simulink model "Mining_Loader_Sweep"  (R2026a)
settings: Solver=ode23t  StopTime=stopTime  AbsTol=1e-3
PostLoadFcn:
  | [extInput_Mining_Loader_Sweep, minMachParams, Init] = test_MLSweep_braking('Mining_Loader_Sweep',minMachParams,testSettings,Init,5,0,0,0,0,0,40);
undefined symbols (not defined in the file): bucketLoadMass, minMachParams, targetSpeedMag, testSettings
libraries: sm_mining_loader_lib x1, simulink_extras x1
settings Model: Creator=gabri  LastModifiedBy=smiller
settings SolverCC: MaxConsecutiveMinStep=5
settings DataIOCC: ExternalInput=extInput_Mining_Loader_Sweep  LoadExternalInput=on  SignalLoggingName=logsout_Mining_Loader_Sweep
settings DebuggingCC: AlgebraicLoopMsg=error
settings SimscapeCC: SimscapeNominalValues="[{\"value\":\"1\",\"unit\":\"A\"},{\"value\":\"1\",\"unit\":\"bar\"},{\"value\":\"1\",\"unit\":\"cm^2\"},{\"value\":\"1\",\"unit\":\"cm^3/s\"},{\"value\":\"1\",\"unit\":\"kJ/kg\"},{\"value\":\"1\",\"unit\":\"kW\"},{\"value\":\"1\",\"unit\":\"l\"},{\"value\":\"1\",\"unit\":\"N\"},{\"value\":\"1\",\"unit\":\"N*m\"},{\"value\":\"1\",\"unit\":\"V\"}]"  SimscapeLogName=simlog_Mining_Loader_Sweep  SimscapeLogLimitData=off  SimscapeLogDataHistory=5000.0
settings DiagnosticsConfigSet: SimMechanicsConflictingReferenceFrames=none
settings ExplorerConfigSet: InternalSimMechanicsExplorerSettings="<ExplorerConfiguration><canonicalview>default</canonicalview><TilePanel><TileInfo><Tiles Columns=\"1\" Count=\"1\" Height=\"438\" Rows=\"1\" Width=\"828\"><Row Weight=\"1\"/><Column Weight=\"1\"/><Tile Height=\"1\" Width=\"1\" X=\"0\" Y=\"0\"/></Tiles></TileInfo><SceneInfo><SceneViewer><IsThisViewStd><IsStandardView>off</IsStandardView><StandardViewName>Front</StandardViewName></IsThisViewStd><BGColor><R>1</R><G>1</G><B>1</B><A>1</A></BGColor><Camera><DoPerspective>on</DoPerspective><Position><X>-19.655173879230539</X><Y>-9.0222687540439601</Y><Z>-1.8989073435199815</Z></Position><Center><X>-19.622924303554189</X><Y>-8.0228109525652247</Y><Z>-1.892268975347827</Z></Center><Up><X>-0.00021408927402311921</X><Y>-0.0066349150538512255</Y><Z>0.99997796579125231</Z></Up><XLim>0.46630765815499881</XLim><YLim>0.46630765815499881</YLim><ViewLimDist>0.01</ViewLimDist></Camera></SceneViewer></SceneInfo></TilePanel><MechEditorPanel><GfxPanelCameraMap><MapElement CameraMLId=\"Camera10\" GfxPanelIndex=\"0\"/></GfxPanelCameraMap><Cameras><Camera><Id>Camera1</Id><Value><Name>Track LR</Name><NativeCamera><PositionTrackingFeature>Mining_Loader.Vehicle.Camera_Frames_R.Cam_Ref_LR.R</PositionTrackingFeature><CenterTrackingFeature>Mining_Loader.Vehicle.Camera_Frames_R.Cam_Ref_Ctr.R</CenterTrackingFeature><UpVectorTrackingFeature>Mining_Loader.World_Frame.W</UpVectorTrackingFeature><CenterTrackingOrigin>on</CenterTrackingOrigin><UpVectorTrackingDirection>+Z</UpVectorTrackingDirection></NativeCamera></Value></Camera><Camera><Id>Camera2</Id><Value><Name>Track RR</Name><NativeCamera><PositionTrackingFeature>Mining_Loader.Vehicle.Camera_Frames_R.Cam_Ref_RR.R</PositionTrackingFeature><CenterTrackingFeature>Mining_Loader.Vehicle.Camera_Frames_R.Cam_Ref_Ctr.R</CenterTrackingFeature><UpVectorTrackingFeature>Mining_Loader.World_Frame.W</UpVectorTrackingFeature><CenterTrackingOrigin>on</CenterTrackingOrigin><UpVectorTrackingDirection>+Z</UpVectorTrackingDirection></NativeCamera></Value></Camera><Camera><Id>Camera3</Id><Value><Name>Track FL</Name><NativeCamera><PositionTrackingFeature>Mining_Loader.Vehicle.Camera_Frames_F.Cam_Ref_FL.R</PositionTrackingFeature><CenterTrackingFeature>Mining_Loader.Vehicle.Camera_Frames_F.Cam_Ref_Ctr.R</CenterTrackingFeature><UpVectorTrackingFeature>Mining_Loader.World_Frame.W</UpVectorTrackingFeature><CenterTrackingOrigin>on</CenterTrackingOrigin><UpVectorTrackingDirection>+Z</UpVectorTrackingDirection></NativeCamera></Value></Camera><Camera><Id>Camera4</Id><Value><Name>Track FR</Name><NativeCamera><PositionTrackingFeature>Mining_Loader.Vehicle.Camera_Frames_F.Cam_Ref_FR.R</PositionTrackingFeature><CenterTrackingFeature>Mining_Loader.Vehicle.Camera_Frames_F.Cam_Ref_Ctr.R</CenterTrackingFeature><UpVectorTrackingFeature>Mining_Loader.World_Frame.W</UpVectorTrackingFeature><CenterTrackingOrigin>on</CenterTrackingOrigin><UpVectorTrackingDirection>+Z</UpVectorTrackingDirection></NativeCamera></Value></Camera><Camera><Id>Camera5</Id><Value><Name>Track Frame Right</Name><NativeCamera><PositionTrackingFeature>Mining_Loader.Vehicle.Camera_Frames_F.Cam_Ref_Right.R</PositionTrackingFeature><CenterTrackingFeature>Mining_Loader.Vehicle.Camera_Frames_F.Cam_Ref_Right.R</CenterTrackingFeature><UpVectorTrackingFeature>Mining_Loader.World_Frame.W</UpVectorTrackingFeature><CenterTrackingOrigin>off</CenterTrackingOrigin><CenterTrackingDirection>-Y</CenterTrackingDirection><UpVectorTrackingDirection>+Z</UpVectorTrackingDirection></NativeCamera></Value></Camera><Camera><Id>Camera6</Id><Value><Name>Track Frame Left</Name><NativeCamera><PositionTrackingFeature>Mining_Loader.Vehicle.Camera_Frames_F.Cam_Ref_Left.R</PositionTrackingFeature><CenterTrackingFeature>Mining_Loader.Vehicle.Camera_Frames_F.Cam_Ref_Left.R</CenterTrackingFeature><UpVectorTrackingFeature>Mining_Loader.World_Frame.W</UpVectorTrackingFeature><CenterTrackingOrigin>off</CenterTrackingOrigin><CenterTrackingDirection>+Y</CenterTrackingDirection><UpVectorTrackingDirection>+Z</UpVectorTrackingDirection></NativeCamera></Value></Camera><Camera><Id>Camera7</Id><Value><Name>Track Frame Top Down</Name><NativeCamera><PositionTrackingFeature>Mining_Loader.Vehicle.Camera_Frames_F.Cam_Ref_Top_Down.R</PositionTrackingFeature><CenterTrackingFeature>Mining_Loader.Vehicle.Camera_Frames_F.Cam_Ref_Top_Down.R</CenterTrackingFeature><UpVectorTrackingFeature>Mining_Loader.Vehicle.Camera_Frames_F.Cam_Ref_Top_Down.R</UpVectorTrackingFeature><CenterTrackingOrigin>off</CenterTrackingOrigin><CenterTrackingDirection>-Z</CenterTrackingDirection><UpVectorTrackingDirection>+Y</UpVectorTrackingDirection></NativeCamera></Value></Camera><Camera><Id>Camera8</Id><Value><Name>Track Frame Rear Fwd</Name><NativeCamera><PositionTrackingFeature>Mining_Loader.Vehicle.Camera_Frames_F.Cam_Ref_Top_Rear_Fwd.R</PositionTrackingFeature><CenterTrackingFeature>Mining_Loader.Vehicle.Camera_Frames_F.Cam_Ref_Top_Rear_Fwd.R</CenterTrackingFeature><UpVectorTrackingFeature>Mining_Loader.World_Frame.W</UpVectorTrackingFeature><CenterTrackingOrigin>off</CenterTrackingOrigin><CenterTrackingDirection>+X</CenterTrackingDirection><UpVectorTrackingDirection>+Z</UpVectorTrackingDirection></NativeCamera></Value></Camera><Camera><Id>Camera9</Id><Value><Name>Track Chassis Right</Name><NativeCamera><PositionTrackingFeature>Mining_Loader.Vehicle.Camera_Frames_R.Cam_Ref_Right.R</PositionTrackingFeature><CenterTrackingFeature>Mining_Loader.Vehicle.Camera_Frames_R.Cam_Ref_Right.R</CenterTrackingFeature><UpVectorTrackingFeature>Mining_Loader.World_Frame.W</UpVectorTrackingFeature><CenterTrackingOrigin>off</CenterTrackingOrigin><CenterTrackingDirection>-Y</CenterTrackingDirection><UpVectorTrackingDirection>+Z</UpVectorTrackingDirection></NativeCamera></Value></Camera><Camera><Id>Camera10</Id><Value><Name>Track Chassis Left</Name><NativeCamera><PositionTrackingFeature>Mining_Loader.Vehicle.Camera_Frames_F.Cam_Ref_Left.R</PositionTrackingFeature><CenterTrackingFeature>Mining_Loader.Vehicle.Camera_Frames_F.Cam_Ref_Left.R</CenterTrackingFeature><UpVectorTrackingFeature>Mining_Loader.World_Frame.W</UpVectorTrackingFeature><CenterTrackingOrigin>off</CenterTrackingOrigin><CenterTrackingDirection>+Y</CenterTrackingDirection><UpVectorTrackingDirection>+Z</UpVectorTrackingDirection></NativeCamera></Value></Camera><Camera><Id>Camera11</Id><Value><Name>Track Chassis Top Down</Name><NativeCamera><PositionTrackingFeature>Mining_Loader.Vehicle.Camera_Frames_R.Cam_Ref_Top_Down.R</PositionTrackingFeature><CenterTrackingFeature>Mining_Loader.Vehicle.Camera_Frames_R.Cam_Ref_Top_Down.R</CenterTrackingFeature><UpVectorTrackingFeature>Mining_Loader.Vehicle.Camera_Frames_R.Cam_Ref_Top_Down.R</UpVectorTrackingFeature><CenterTrackingOrigin>off</CenterTrackingOrigin><CenterTrackingDirection>-Z</CenterTrackingDirection><UpVectorTrackingDirection>+Y</UpVectorTrackingDirection></NativeCamera></Value></Camera><Camera><Id>Camera12</Id><Value><Name>Track Chassis Rear Fwd</Name><NativeCamera><PositionTrackingFeature>Mining_Loader.Vehicle.Camera_Frames_R.Cam_Ref_Top_Rear_Fwd.R</PositionTrackingFeature><CenterTrackingFeature>Mining_Loader.Vehicle.Camera_Frames_R.Cam_Ref_Top_Rear_Fwd.R</CenterTrackingFeature><UpVectorTrackingFeature>Mining_Loader.World_Frame.W</UpVectorTrackingFeature><CenterTrackingOrigin>off</CenterTrackingOrigin><CenterTrackingDirection>+X</CenterTrackingDirection><UpVectorTrackingDirection>+Z</UpVectorTrackingDirection></NativeCamera></Value></Camera></Cameras><VideoCreator><IncludeTiles>All</IncludeTiles><IncludeTime>on</IncludeTime><IncludeWorldFrame>off</IncludeWorldFrame><PlaybackSpeedRatio>1</PlaybackSpeedRatio><FrameRate>30</FrameRate><FrameSize>auto</FrameSize><VideoFormat>UncompressedAVI</VideoFormat></VideoCreator></MechEditorPanel><PlaybackSettings><PlaybackSpeedFactor>8</PlaybackSpeedFactor></PlaybackSettings></ExplorerConfiguration>"

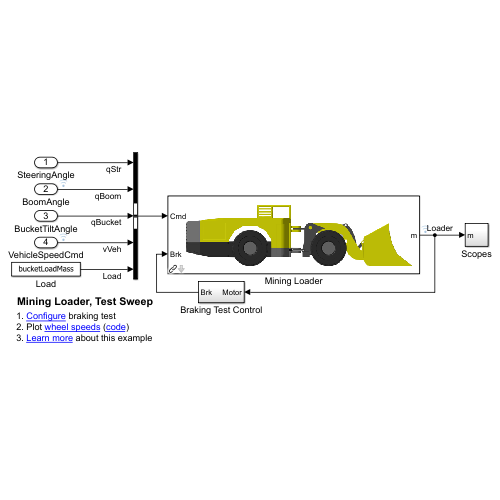
[thumbnail: Simulink's stored preview of the top-level diagram]
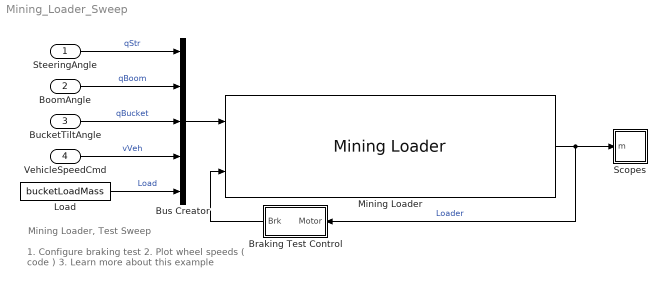
== system Mining_Loader_Sweep ==
  note: Mining Loader, Test Sweep
  note: 1. Configure braking test
      | 2. Plot wheel speeds ( code )
      | 3. Learn more about this example
  SteeringAngle : Inport
  BoomAngle : Inport  Port=2
  BucketTiltAngle : Inport  Port=3
  VehicleSpeedCmd : Inport  Port=4
  Braking Test Control : Subsystem
  Bus Creator : BusCreator  Inputs=5
  Load : Constant  Value=bucketLoadMass
  Mining Loader : sm_mining_loader_lib/Mining Loader  popup_steer_actuation=Hinge Motion  popup_lift_actuation=Hinge Motion  popup_tilt_actuation=Hinge Motion  popup_scene=SlopeX  popup_sensor=None
  Scopes : Subsystem
  wires:
  BucketTiltAngle/1 -> Bus Creator/3  "qBucket"
  BoomAngle/1 -> Bus Creator/2  "qBoom"
  SteeringAngle/1 -> Bus Creator/1  "qStr"
  VehicleSpeedCmd/1 -> Bus Creator/4  "vVeh"
  Bus Creator/1 -> Mining Loader/1
  Mining Loader/1 -> Braking Test Control/1(Motor), Scopes/1(m)  "Loader"
  Braking Test Control/1(Brk) -> Mining Loader/2
  Load/1 -> Bus Creator/5  "Load"

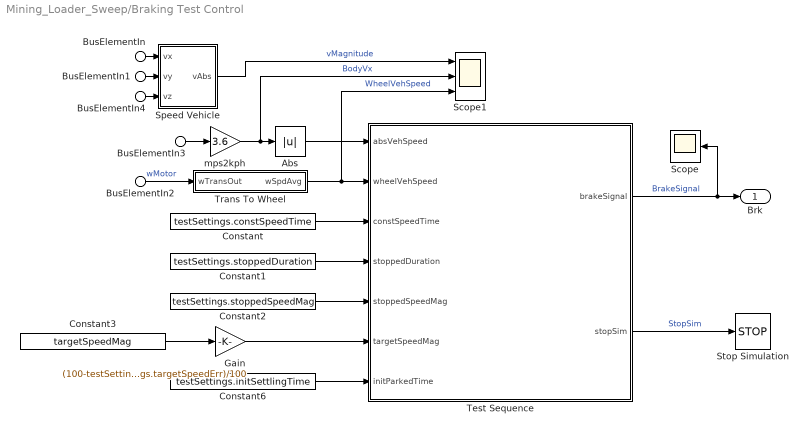
== system Mining_Loader_Sweep/Braking Test Control ==
  BusElementIn : Inport  PortName=Motor  Element=World.vx
  BusElementIn1 : Inport  PortName=Motor  Element=World.vy
  BusElementIn4 : Inport  PortName=Motor  Element=World.vz
  BusElementIn2 : Inport  PortName=Motor  Element=Trans.wOut
  BusElementIn3 : Inport  PortName=Motor  Element=Vehicle.Frame.Body.vx
  Abs : Abs  ZeroCross=off  SaturateOnIntegerOverflow=off
  Constant : Constant  Value=testSettings.constSpeedTime
  Constant1 : Constant  Value=testSettings.stoppedDuration
  Constant2 : Constant  Value=testSettings.stoppedSpeedMag
  Constant3 : Constant  Value=targetSpeedMag
  Constant6 : Constant  Value=testSettings.initSettlingTime
  Gain : Gain  Gain=(100-testSettings.targetSpeedErr)/100
  Scope : Scope
      settings: ActiveDisplayYMinimum=-0.12499999999999997  ActiveDisplayYMaximum=1.125  DataLoggingVariableName=ScopeData4
  Scope1 : Scope  NumInputPorts=3
      settings: ActiveDisplayYMinimum=-15.003580591871296  ActiveDisplayYMaximum=14.898540881762012
  Speed Vehicle : Subsystem
  Stop Simulation : Stop
  Test Sequence : Stateflow chart  TreatAsAtomicUnit=on
      settings: PortSchema="{\"entries\":[{\"content\":{\"sides\":[{\"content\":{\"connectorIds\":[\"In2\",\"In1\",\"In3\",\"In4\",\"In5\",\"In6\",\"In7\"]},\"type\":\"ConnectorPlacement.EquallySpacedRectSide\",\"uuid\":\"e1937b18-ff72-43a3-acf8-9fe8c933d130\"},{\"content\":{\"connectorIds\":[\"Out1\",\"Out2\"],\"side\":\"RIGHT\"},\"type\":\"ConnectorPlacement.EquallySpacedRectSide\",\"uuid\":\"ae5e9681-f55f-479e-9a9a-2b26d8d878fe\"},{\"content\":{\"side\":\"TOP\"},\"type\":\"ConnectorPlacement.EquallySpacedRectSide\",\"uuid\":\"437c0b29-f875-47eb-a595-1752e0995e58\"}]},\"type\":\"ConnectorPlacement.EquallySpacedConnector\",\"uuid\":\"b3ca529e-f5d1-4eb0-8354-141722a10c74\"}],\"packageUris\":[\"http://schema.mathworks.com/mf0/Connector/R2020b\"],\"version\":\"1.0\"}"
  Trans To Wheel : Subsystem
  mps2kph : Gain  Gain=3.6
  Brk : Outport
  wires:
  Abs/1 -> Test Sequence/2(absVehSpeed)
  Test Sequence/2(stopSim) -> Stop Simulation/1  "StopSim"
  Constant/1 -> Test Sequence/3(constSpeedTime)
  Constant2/1 -> Test Sequence/5(stoppedSpeedMag)
  Constant1/1 -> Test Sequence/4(stoppedDuration)
  Test Sequence/1(brakeSignal) -> Scope/1, Brk/1  "BrakeSignal"
  Constant3/1 -> Gain/1
  Gain/1 -> Test Sequence/6(targetSpeedMag)
  Constant6/1 -> Test Sequence/7(initParkedTime)
  Trans To Wheel/1(wSpdAvg) -> Scope1/3, Test Sequence/1(wheelVehSpeed)  "WheelVehSpeed"
  BusElementIn2/1 -> Trans To Wheel/1(wTransOut)  "wMotor"
  BusElementIn4/1 -> Speed Vehicle/3(vz)
  BusElementIn1/1 -> Speed Vehicle/2(vy)
  BusElementIn/1 -> Speed Vehicle/1(vx)
  BusElementIn3/1 -> mps2kph/1
  mps2kph/1 -> Scope1/2, Abs/1  "BodyVx"
  Speed Vehicle/1(vAbs) -> Scope1/1  "vMagnitude"

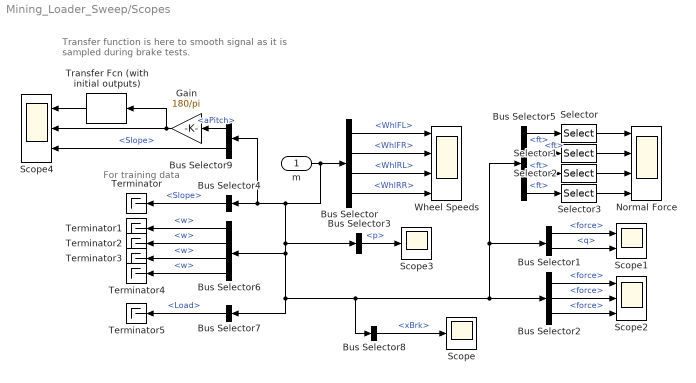
== system Mining_Loader_Sweep/Scopes ==
  note: Transfer function is here to smooth signal as it is sampled during brake tests.
  note: For training data
  m : Inport
  Bus Selector : BusSelector  OutputSignals=Vehicle.Frame.WhlFL,Vehicle.Frame.WhlFR,Vehicle.Chassis.WhlRL,Vehicle.Chassis.WhlRR
  Bus Selector1 : BusSelector  OutputSignals=Vehicle.Steer.L.force,Vehicle.Steer.H.q
  Bus Selector2 : BusSelector  OutputSignals=Vehicle.Steer.L.force,Vehicle.Lift.L.force,Vehicle.Tilt.A.force
  Bus Selector3 : BusSelector  OutputSignals=Vehicle.Steer.L.p
  Bus Selector4 : BusSelector  OutputSignals=Scene.Slope
  Bus Selector5 : BusSelector  OutputSignals=Vehicle.Frame.TireFL.ft,Vehicle.Frame.TireFR.ft,Vehicle.Chassis.TireRL.ft,Vehicle.Chassis.TireRR.ft
  Bus Selector6 : BusSelector  OutputSignals=Vehicle.Frame.WhlFL.w,Vehicle.Frame.WhlFR.w,Vehicle.Chassis.WhlRL.w,Vehicle.Chassis.WhlRR.w
  Bus Selector7 : BusSelector  OutputSignals=Vehicle.Bucket.Load
  Bus Selector8 : BusSelector  OutputSignals=Sensor.xBrk
  Bus Selector9 : BusSelector  OutputSignals=World.aPitch,Scene.Slope
  Gain : Gain  Gain=180/pi
  Normal Force : Scope  NumInputPorts=4
      settings: ActiveDisplayYMinimum=-34779.002353913609  ActiveDisplayYMaximum=313011.02118522255  DataLoggingVariableName=ScopeData6
  Scope : Scope
      settings: ActiveDisplayYMinimum=-0.65988877092317455  ActiveDisplayYMaximum=5.8947656760621783  DataLoggingVariableName=ScopeData10
  Scope1 : Scope  NumInputPorts=2
      settings: ActiveDisplayYMinimum=-1  ActiveDisplayYMaximum=1  DataLoggingVariableName=ScopeData2
  Scope2 : Scope  NumInputPorts=3
      settings: ActiveDisplayYMinimum=-1  ActiveDisplayYMaximum=1  DataLoggingVariableName=ScopeData3
  Scope3 : Scope
      settings: ActiveDisplayYMinimum=-1  ActiveDisplayYMaximum=1  DataLoggingVariableName=ScopeData5
  Scope4 : Scope  NumInputPorts=3
      settings: ActiveDisplayYMinimum=-12.327016669989776  ActiveDisplayYMaximum=-9.1542521016721565  DataLoggingVariableName=ScopeData8
  Selector{,1..3} (4 alike) : Selector  InputPortWidth=3  IndexOptions=Index vector (dialog)  Indices=[3]  OutputSizes=1
  Terminator{,1..5} (6 alike) : Terminator
  Transfer Fcn (with initial outputs) : simulink_extras/Additional Linear/Transfer Fcn (with initial outputs)  N=[1]  D="[1  1]"  Y0=Init.Vehicle.pitch  U0=Init.Vehicle.pitch
  Wheel Speeds : Scope  NumInputPorts=4
      settings: ActiveDisplayYMinimum=-3.8834266281494827  ActiveDisplayYMaximum=0.12495994005614847
  wires:
  m/1 -> Bus Selector6/1, Bus Selector8/1, Bus Selector5/1, Bus Selector1/1, Bus Selector2/1, Bus Selector7/1, Bus Selector3/1, Bus Selector9/1, Bus Selector4/1, Bus Selector/1
  Bus Selector/2 -> Wheel Speeds/2  "<WhlFR>"
  Bus Selector/3 -> Wheel Speeds/3  "<WhlRL>"
  Bus Selector/4 -> Wheel Speeds/4  "<WhlRR>"
  Bus Selector1/1 -> Scope1/1  "<force>"
  Bus Selector1/2 -> Scope1/2  "<q>"
  Bus Selector2/2 -> Scope2/2  "<force>"
  Bus Selector2/3 -> Scope2/3  "<force>"
  Bus Selector3/1 -> Scope3/1  "<p>"
  Bus Selector2/1 -> Scope2/1  "<force>"
  Bus Selector4/1 -> Terminator/1  "<Slope>"
  Bus Selector/1 -> Wheel Speeds/1  "<WhlFL>"
  Bus Selector6/1 -> Terminator1/1  "<w>"
  Bus Selector6/2 -> Terminator2/1  "<w>"
  Bus Selector6/3 -> Terminator3/1  "<w>"
  Bus Selector6/4 -> Terminator4/1  "<w>"
  Bus Selector7/1 -> Terminator5/1  "<Load>"
  Bus Selector5/1 -> Selector/1  "<ft>"
  Bus Selector5/2 -> Selector1/1  "<ft>"
  Bus Selector5/3 -> Selector2/1  "<ft>"
  Bus Selector5/4 -> Selector3/1  "<ft>"
  Selector/1 -> Normal Force/1
  Selector1/1 -> Normal Force/2
  Selector2/1 -> Normal Force/3
  Selector3/1 -> Normal Force/4
  Bus Selector8/1 -> Scope/1  "<xBrk>"
  Bus Selector9/1 -> Gain/1  "<aPitch>"
  Bus Selector9/2 -> Scope4/3  "<Slope>"
  Gain/1 -> Transfer Fcn (with initial outputs)/1, Scope4/2
  Transfer Fcn (with initial outputs)/1 -> Scope4/1

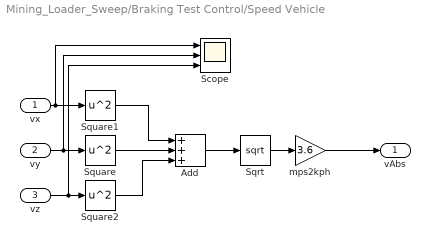
== system Mining_Loader_Sweep/Braking Test Control/Speed Vehicle ==
  vx : Inport
  vy : Inport  Port=2
  vz : Inport  Port=3
  Add : Sum  Inputs=+++
  Scope : Scope  NumInputPorts=3
      settings: ActiveDisplayYMinimum=-0.17801645642040786  ActiveDisplayYMaximum=0.24277511899293014  DataLoggingVariableName=ScopeData7
  Sqrt : Sqrt
  Square : Math  Operator=square
  Square1 : Math  Operator=square
  Square2 : Math  Operator=square
  mps2kph : Gain  Gain=3.6
  vAbs : Outport
  wires:
  Square1/1 -> Add/1
  Add/1 -> Sqrt/1
  vz/1 -> Scope/3, Square2/1
  Square/1 -> Add/2
  Square2/1 -> Add/3
  Sqrt/1 -> mps2kph/1
  vx/1 -> Scope/1, Square1/1
  vy/1 -> Scope/2, Square/1
  mps2kph/1 -> vAbs/1

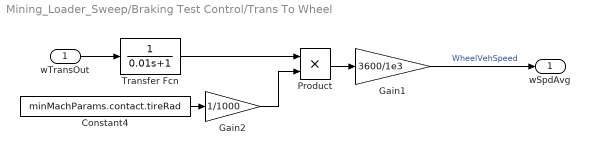
== system Mining_Loader_Sweep/Braking Test Control/Trans To Wheel ==
  wTransOut : Inport
  Constant4 : Constant  Value=minMachParams.contact.tireRad
  Gain1 : Gain  Gain=3600/1e3
  Gain2 : Gain  Gain=1/1000
  Product : Product
  Transfer Fcn : TransferFcn  Denominator=[0.01 1]
  wSpdAvg : Outport
  wires:
  Transfer Fcn/1 -> Product/1
  Product/1 -> Gain1/1
  Gain1/1 -> wSpdAvg/1  "WheelVehSpeed"
  Gain2/1 -> Product/2
  wTransOut/1 -> Transfer Fcn/1
  Constant4/1 -> Gain2/1

== stateflow chart Mining_Loader_Sweep/Braking Test Control/Test Sequence ==
  state Initialization
    entry:
    brakeSignal = 1;
    stopSim = 0;
  state StopSim
    entry:
    stopSim = 1;
  state NotAtTarget
    entry:
    brakeSignal = 0;
  state AtTarget
  state EngageBrake
    entry:
    brakeSignal=1;
  (default) -> Initialization
  EngageBrake -> StopSim : [duration(absVehSpeed<=stoppedSpeedMag) > stoppedDuration]
  Initialization -> NotAtTarget : [after(initParkedTime,'sec')]
  NotAtTarget -> AtTarget : [abs(wheelVehSpeed)>=targetSpeedMag]
  AtTarget -> EngageBrake : [after(constSpeedTime,'sec')]
  data: wheelVehSpeed input; absVehSpeed input; brakeSignal output double; stopSim output double; constSpeedTime input; stoppedDuration input; stoppedSpeedMag input; targetSpeedMag input; initParkedTime input
